simulink subsystem "StudentTemplate_SNGKHA008_M2_Prac"  (R2025b)
settings: Solver=VariableStepAuto  StartTime=0.0  StopTime=10.0  RelTol=1e-3
libraries: simulink x5
settings Model: Creator=JesseJabezArendse  LastModifiedBy=muner

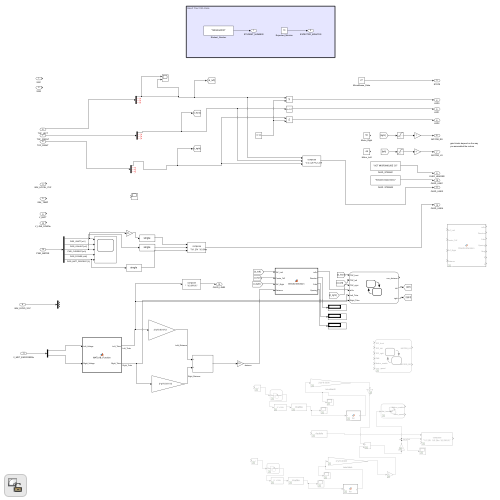
[thumbnail: Simulink's stored preview of the top-level diagram]
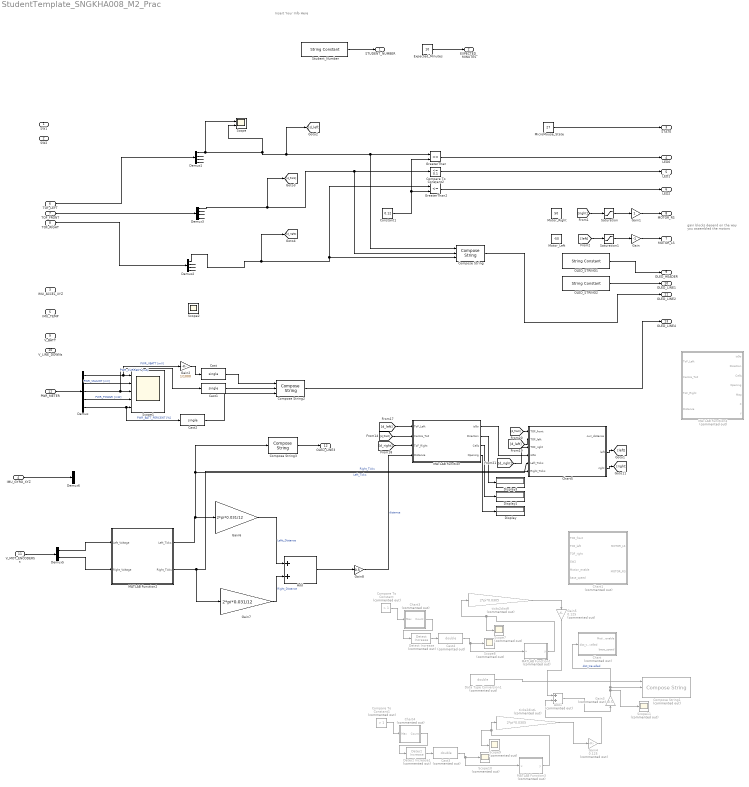
== system StudentTemplate_SNGKHA008_M2_Prac ==
  note: gain blocks depend on the way
      | you assembled the motors
  note: Insert Your Info Here
  SW1 : Inport
  SW2 : Inport  Port=2
  IMU_ACCEL_XYZ : Inport  Port=3
  IMU_GYRO_XYZ : Inport  Port=4
  IMU_TEMP : Inport  Port=5
  TOF_LEFT : Inport  Port=6
  TOF_FRONT : Inport  Port=7
  TOF_RIGHT : Inport  Port=8
  V_BATT : Inport  Port=9
  V_LINE_DOWNs : Inport  Port=10
  V_MOT_ENCODERSs : Inport  Port=11
  PWR_METER : Inport  Port=12
  Add : Sum
  Add1 : Sum  Commented=on
  Cast : DataTypeConversion  OutDataTypeStr=single  SaturateOnIntegerOverflow=off  RndMeth=Floor
  Cast1 : DataTypeConversion  OutDataTypeStr=single  SaturateOnIntegerOverflow=off  RndMeth=Floor
  Cast2 : DataTypeConversion  OutDataTypeStr=single  SaturateOnIntegerOverflow=off  RndMeth=Floor
  Cast3 : DataTypeConversion  Commented=on  OutDataTypeStr=double  SaturateOnIntegerOverflow=off  RndMeth=Floor
  Cast4 : DataTypeConversion  Commented=on  OutDataTypeStr=double  SaturateOnIntegerOverflow=off  RndMeth=Floor
  Chart : Stateflow chart  Commented=on  TreatAsAtomicUnit=on
  Chart1 : Stateflow chart  Commented=on  TreatAsAtomicUnit=on
  Chart3 : Stateflow chart  Commented=on  TreatAsAtomicUnit=on
  Chart4 : Stateflow chart  Commented=on  TreatAsAtomicUnit=on
  Chart5 : Stateflow chart  TreatAsAtomicUnit=on
  Compare To Constant : simulink/Logic and Bit Operations/Compare To Constant  Commented=on  relop=>  const=1  OutDataTypeStr=boolean
  Compare To Constant1 : simulink/Logic and Bit Operations/Compare To Constant  Commented=on  relop=>  const=1  OutDataTypeStr=boolean
  Compare To Constant2 : simulink/Logic and Bit Operations/Compare To Constant  relop=<=  const=0.1  OutDataTypeStr=boolean
  Compose String : ComposeString  Format="\"L%1.2f F%1.2f R%1.2f\""
  Compose String1 : ComposeString  Commented=on  Format="\"%1.2fV  %3.2fm  %2.0f%%\""
  Compose String2 : ComposeString  Format="\"%1.2fV  %3.0fmA  %2.0f%%\""
  Compose String3 : ComposeString  Format="\"  %3.0f%%\""
  Constant1 : Constant  Value=0.12  SampleTime=-1
  Data Type Conversion1 : DataTypeConversion  Commented=on  OutDataTypeStr=double  SaturateOnIntegerOverflow=off  RndMeth=Floor
  Demux : Demux  Outputs=5
  Demux1 : Demux
  Demux2 : Demux
  Demux3 : Demux
  Demux5 : Demux  Outputs=2
  Demux6 : Demux  Outputs=3
  Detect Increase : simulink/Logic and Bit Operations/Detect Increase  Commented=on  vinit=0.0  OutDataTypeStr=boolean
  Detect Increase1 : simulink/Logic and Bit Operations/Detect Increase  Commented=on  vinit=0.0  OutDataTypeStr=boolean
  Display : Display
  Display1 : Display
  Display3 : Display
  Expected_Minutes : Constant  Value=10  OutDataTypeStr=uint8
  Gain : Gain  Gain=-1  OutDataTypeStr=Inherit: Same as input
  Gain1 : Gain  OutDataTypeStr=Inherit: Same as input
  Gain2 : Gain  Gain=1/1000
  Gain3 : Gain  Commented=on  Gain=0.5
  Gain4 : Gain  Commented=on  Gain=0.125
  Gain5 : Gain  Commented=on  Gain=0.125
  Gain6 : Gain  Gain=2*pi*0.031/12
  Gain7 : Gain  Gain=2*pi*0.031/12
  Gain8 : Gain  Gain=0.5  OutDataTypeStr=double
  GreaterThan : RelationalOperator  Operator=<=  OutDataTypeStr=boolean  RndMeth=Simplest  InputSameDT=off
  GreaterThan2 : RelationalOperator  Operator=<=  OutDataTypeStr=boolean  RndMeth=Simplest  InputSameDT=off
  MATLAB Function : MATLAB Function  TreatAsAtomicUnit=on
  MATLAB Function1 : MATLAB Function  Commented=on  TreatAsAtomicUnit=on
  MATLAB Function2 : MATLAB Function  TreatAsAtomicUnit=on
  MATLAB Function3 : MATLAB Function  Commented=on  TreatAsAtomicUnit=on
  MATLAB Function4 : MATLAB Function  Commented=on  TreatAsAtomicUnit=on
  MicroMouse_State : Constant  Value=27
  Motor_Left : Constant  Value=-50
  Motor_Right : Constant  Value=50
  OLED_STRING1 : StringConstant  String="\"UCT MICROMOUSE '25\""
  OLED_STRING2 : StringConstant  String="\"Simulink Data Demo\""
  Saturation : Saturate  UpperLimit=100  LowerLimit=-100
  Saturation1 : Saturate  UpperLimit=100  LowerLimit=-100
  Scope : Scope  NumInputPorts=2
      settings: ActiveDisplayYMinimum=0.22759  ActiveDisplayYMaximum=0.52326  DataLoggingVariableName=ScopeData5
  Scope1 : Scope  NumInputPorts=5
      settings: ActiveDisplayYMinimum=-437.5  ActiveDisplayYMaximum=3937.5  DataLoggingVariableName=ScopeData6
  Scope{7..11} (5 alike) : Scope  Commented=on
      Scope10 settings: ActiveDisplayYMinimum=-1.0332830006305334  ActiveDisplayYMaximum=1.171716999369468
      Scope11 settings: DataLoggingVariableName=ScopeData12
      Scope7 settings: ActiveDisplayYMinimum=34.194505967509976  ActiveDisplayYMaximum=50.493839833256565  DataLoggingVariableName=ScopeData10
      Scope8 settings: ActiveDisplayYMinimum=-1.0332830006305334  ActiveDisplayYMaximum=1.171716999369468  DataLoggingVariableName=ScopeData11
      Scope9 settings: ActiveDisplayYMinimum=34.194505967509976  ActiveDisplayYMaximum=50.493839833256565  DataLoggingVariableName=ScopeData2
  Scope2 : Scope
  Student_Number : StringConstant  String="\"SNGKHA008\""
  ticks2distL : Gain  Commented=on  Gain=2*pi*0.0305
  ticks2distR : Gain  Commented=on  Gain=2*pi*0.0305
  STUDENT_NUMBER : Outport
  EXPECTED_MINUTES : Outport  Port=2
  STATE : Outport  Port=3
  LED0 : Outport  Port=4
  LED1 : Outport  Port=5
  LED2 : Outport  Port=6
  MOTOR_LS : Outport  Port=7
  MOTOR_RS : Outport  Port=8
  OLED_HEADER : Outport  Port=9
  OLED_LINE1 : Outport  Port=10
  OLED_LINE2 : Outport  Port=11
  OLED_LINE3 : Outport  Port=12
  OLED_LINE4 : Outport  Port=13
  wires:
  TOF_FRONT/1 -> Demux3/1
  OLED_STRING2/1 -> OLED_LINE1/1
  Demux2/3 -> ?
  Demux2/2 -> ?
  Demux2/4 -> ?
  Compare To Constant2/1 -> LED1/1
  Demux3/3 -> ?
  TOF_RIGHT/1 -> Demux2/1
  Demux3/4 -> ?
  Demux3/2 -> ?
  Demux1/2 -> ?
  OLED_STRING1/1 -> OLED_HEADER/1
  Compose String/1 -> OLED_LINE2/1
  Constant1/1 -> GreaterThan2/2, GreaterThan/2
  Demux1/4 -> ?
  TOF_LEFT/1 -> Demux1/1
  Demux1/3 -> ?
  PWR_METER/1 -> Demux/1
  Demux/1 -> Scope1/1, Gain2/1  "PWR_VBATT [mV]"
  Demux/2 -> Scope1/2  "PWR_VSHUNT [mV]"
  Demux/3 -> Scope1/3, Cast1/1  "PWR_CURRENT [mA]"
  Demux/4 -> Scope1/4  "PWR_POWER [mW]"
  Demux/5 -> Scope1/5, Cast2/1  "PWR_BATT_PERCENT [%]"
  Compose String2/1 -> OLED_LINE4/1
  Gain2/1 -> Cast/1
  Cast/1 -> Compose String2/1
  Cast1/1 -> Compose String2/2
  Cast2/1 -> Compose String2/3
  Demux2/1 -> Compose String/3, GreaterThan2/1, [d_right]
  Demux1/1 -> Scope/1, Scope/2, Compose String/1, GreaterThan/1, [d_left]
  MicroMouse_State/1 -> STATE/1
  Student_Number/1 -> STUDENT_NUMBER/1
  Expected_Minutes/1 -> EXPECTED_MINUTES/1
  V_MOT_ENCODERSs/1 -> Demux5/1
  [right] -> Saturation/1
  [left] -> Saturation1/1
  IMU_GYRO_XYZ/1 -> Demux6/1
  GreaterThan/1 -> LED0/1
  GreaterThan2/1 -> LED2/1
  Saturation/1 -> Gain1/1
  Saturation1/1 -> Gain/1
  Gain1/1 -> MOTOR_RS/1
  Gain/1 -> MOTOR_LS/1
  Demux3/1 -> Compose String/2, Compare To Constant2/1, [d_front]
  [d_front] -> MATLAB Function/2(Centre_ToF)
  [d_left] -> MATLAB Function/1(ToF_Left)
  [d_right] -> MATLAB Function/3(ToF_Right)
  Demux5/1 -> MATLAB Function2/1(Left_Voltage)
  Demux5/2 -> MATLAB Function2/2(Right_Voltage)
  Add/1 -> Gain8/1
  Gain6/1 -> Add/1  "Leftt_Distance"
  Gain7/1 -> Add/2  "Right_Distance"
  MATLAB Function2/1(Left_Ticks) -> Gain6/1, Chart5/5(Left_Ticks), Compose String3/1  "Left_Ticks"
  MATLAB Function2/2(Right_Ticks) -> Gain7/1, Chart5/6(Right_Ticks)  "Right_Ticks"
  Gain8/1 -> MATLAB Function/4(Distance)  "distance"
  MATLAB Function/1(isGo) -> Chart5/4(isGo)
  [d_left] -> Chart5/2(TOF_left)
  [d_front] -> Chart5/1(TOF_front)
  [d_right] -> Chart5/3(TOF_right)
  Chart5/3(right) -> [right]
  Chart5/2(left) -> [left]
  MATLAB Function/2(Direction) -> Display3/1
  MATLAB Function/3(Cells) -> Display1/1
  MATLAB Function/4(Opening) -> Display/1
  Compose String3/1 -> OLED_LINE3/1
  Cast3/1 -> MATLAB Function3/1(u), Scope10/1
  MATLAB Function3/1(y) -> Scope9/1, ticks2distL/1
  Add1/1 -> Gain3/1
  MATLAB Function1/1(y) -> Scope7/1, ticks2distR/1
  Gain3/1 -> Chart/1(dist_travelled), Compose String1/2, Scope11/1  "dist_travelled"
  Data Type Conversion1/1 -> Compose String1/1
  Compare To Constant1/1 -> Chart4/1(Max)
  Chart4/1(Count) -> Detect Increase1/1
  Chart3/1(Count) -> Detect Increase/1
  Compare To Constant/1 -> Chart3/1(Max)
  Detect Increase/1 -> Cast4/1
  Gain4/1 -> Add1/2
  Gain5/1 -> Add1/1
  Detect Increase1/1 -> Cast3/1
  ticks2distR/1 -> Gain5/1
  Cast4/1 -> MATLAB Function1/1(u), Scope8/1
  ticks2distL/1 -> Gain4/1

== matlab function StudentTemplate_SNGKHA008_M2_Prac/MATLAB Function4 ==
  data: ToF_Left input; isGo output; Centre_ToF input; ToF_Right input; Distance input; Direction output; Cells output; Opening output; Map output; X output; Y output
function [isGo, Direction, Cells, Opening, Map, X, Y] = DirectionDecision(ToF_Left, Centre_ToF, ToF_Right, Distance)
%#codegen
% Determines the robot's movement direction based on ToF sensor readings
% and maps the maze structure.
%
% Outputs a state trigger 'isGo' for a Stateflow chart.
% Also tracks the current facing direction, cell count, and maze map.
%
% Inputs:
%   ToF_Left, Centre_ToF, ToF_Right : Time-of-Flight sensor readings
%   Distance : Total distance traveled (for cell counting)
%
% Outputs:
%   isGo : Numeric trigger for Stateflow
%       1  -> Straight (Start)
%       2  -> Left Turn (turnleft)
%       3  -> Right Turn (turnright)
%       4  -> U-Turn (uturn)
%   Direction : Numeric value representing current facing direction
%       1  -> North
%       2  -> East  
%       3  -> South
%       4  -> West
%   Cells : Number of visited cells
%   Opening : Opening detection
%       -1  -> Opening on left
%       1   -> Opening on right
%       0   -> No opening detected
%   Map : The maze map (Y, X, Layer)
%         Layer 1: North Wall (0=Unk, 1=Wall, 2=Open)
%         Layer 2: East Wall
%         Layer 3: South Wall
%         Layer 4: West Wall
%         Layer 5: Visited (0=No, 1=Yes)
%   X, Y : Robot's current cell coordinates

% --- Thresholds ---
front_threshold = 0.12;
side_threshold  = 0.12;
opening_threshold = 0.2;  % Threshold for detecting openings
cell_distance = 0.16;     % Assumed distance per cell (meters)
post_turn_dist = 0.10;    % Distance to move after turn to center in cell

% --- Map & Coordinate Constants ---
MAP_SIZE_Y = 30;
MAP_SIZE_X = 30;
WALL_N = 1;
WALL_E = 2;
WALL_S = 3;
WALL_W = 4;
LAYER_VISITED = 5;
MAP_UNKNOWN = 0;
MAP_WALL = 1;
MAP_OPEN = 2;

% --- Persistent variables for state tracking ---
persistent currentDirection lastTurnState
persistent lastDistance distanceOffset
persistent lastOpening
persistent startupTimer startupDelayCompleted
persistent postTurnCooldownDistance

% --- NEW Persistent Map & Coordinate variables ---
persistent mazeMap currentX currentY

% --- Initialize persistent variables ---
if isempty(currentDirection)
    currentDirection = 1; % start facing North
    lastTurnState = 0; % previous turn (0 means no-turn)
    
    lastDistance = Distance;
    distanceOffset = Distance; % Initialize offset to current distance
    
    lastOpening = 0; % Initialize opening to 0
    
    startupTimer = 0; % Initialize startup timer
    startupDelayCompleted = false; % Startup delay not completed
    
    postTurnCooldownDistance = 0.0; % Initialize cooldown to 0
    
    % --- NEW Map Initialization ---
    mazeMap = zeros(MAP_SIZE_Y, MAP_SIZE_X, 5, 'uint8');
    currentX = 15; % Start in middle
    currentY = 15; % Start in middle
    % Mark starting cell as visited
    mazeMap(currentY, currentX, LAYER_VISITED) = 1;
end

% --- Startup Delay Logic ---
if ~startupDelayCompleted
    startupTimer = startupTimer + 1;
    if startupTimer >= 100  % Adjust as needed
        startupDelayCompleted = true;
    end
    
    isGo = 0; % Stay still during startup
    Direction = currentDirection;
    Cells = 0;
    Opening = 0;
    % Output initial map and coords
    Map = mazeMap;
    X = currentX;
    Y = currentY;
    return; % Exit early during startup delay
end

% --- NEW: Update Map for CURRENT Cell ---
% This function updates the walls of the cell (currentY, currentX)
% based on the robot's current direction and sensor readings.
mazeMap = updateCellWalls(mazeMap, currentY, currentX, currentDirection, ...
    ToF_Left, Centre_ToF, ToF_Right, ...
    front_threshold, side_threshold, opening_threshold, ...
    MAP_UNKNOWN, MAP_WALL, MAP_OPEN, ...
    WALL_N, WALL_E, WALL_S, WALL_W);

% --- Decide Turn based on sensors ---
opening_left = (ToF_Left > opening_threshold);
opening_right = (ToF_Right > opening_threshold);
localTurn = 0;
if (Centre_ToF < front_threshold) && (ToF_Left < side_threshold) && (ToF_Right < side_threshold)
    localTurn = 2; % dead-end -> U-turn
elseif (Centre_ToF < front_threshold) && (ToF_Left < side_threshold)
    localTurn = 1; % front+left blocked -> turn right
elseif (Centre_ToF < front_threshold) && (ToF_Right < side_threshold)
    localTurn = -1; % front+right blocked -> turn left
elseif (Centre_Tof < front_threshold)
    if ToF_Left > ToF_Right
        localTurn = -1; % more space on left -> turn left
    else
        localTurn = 1;  % more space on right -> turn right
    end
else
    % Front is OPEN (Centre_ToF >= front_threshold)
    
    % Check if we are in the post-turn cooldown period
    if Distance < postTurnCooldownDistance
        % If yes, FORCE straight to clear the corner
        localTurn = 0;
    else
        % If no cooldown, check for side openings as normal
        if opening_left && opening_right
            if ToF_Left > ToF_Right
                localTurn = -1; % Prefer left
            else
                localTurn = 1;  % Prefer right
            end
        elseif opening_left
            localTurn = -1; % Only left is open, turn left
        elseif opening_right
            localTurn = 1;  % Only right is open, turn right
        else
            localTurn = 0; % No openings, go straight
        end
    end
end

% --- Opening Detection Logic ---
if localTurn == 0
    if opening_left
        lastOpening = -1;
    elseif opening_right
        lastOpening = 1;
    else
        lastOpening = 0;
    end
end
Opening = lastOpening;

% --- Update direction only on the rising edge of a turn ---
if (lastTurnState == 0) && (localTurn ~= 0)
    if localTurn == 1
        delta = 1;  % Right turn
    elseif localTurn == -1
        delta = -1; % Left turn
    elseif localTurn == 2
        delta = 2;  % U-turn
    else
        delta = 0;
    end
    currentDirection = mod((currentDirection - 1) + delta, 4) + 1;
end

% --- MODIFIED BLOCK (Handle Cell Transition after a Turn) ---
% Check if we just completed a turn (transition from non-zero to zero)
if (lastTurnState ~= 0) && (localTurn == 0)
    
    % --- NEW: Update Coordinates ---
    % We have finished a turn and are now entering a new cell
    if lastTurnState ~= 2  % If the last turn was NOT a U-turn
        switch currentDirection
            case 1 % Facing North
                currentY = currentY - 1;
            case 2 % Facing East
                currentX = currentX + 1;
            case 3 % Facing South
                currentY = currentY + 1;
            case 4 % Facing West
                currentX = currentX - 1;
        end
        % Mark the new cell as visited
        mazeMap(currentY, currentX, LAYER_VISITED) = 1;
    end
    
    % Force robot to move straight after a turn
    % to clear the corner before making new decisions.
    postTurnCooldownDistance = Distance + post_turn_dist;
    
    distanceOffset = Distance;
end
% Update lastTurnState AFTER the "completed turn" check
if localTurn == 0
    lastTurnState = 0;
else
    lastTurnState = localTurn; % remember we are in a turn state
end
Direction = currentDirection;

% -------- Cell transition logic (straight corridors) --------
% Count cells based on distance traveled when moving straight
if localTurn == 0
    % Calculate effective distance (ignoring distance during turns)
    effectiveDistance = Distance - distanceOffset;
    
    % Each ~0.16 meters = 1 cell
    if effectiveDistance >= (cell_distance + 0.01) % Add small buffer
        cellsFromDistance = floor(effectiveDistance / cell_distance);
        
        % --- NEW: Update Coords for each cell ---
        for i = 1:cellsFromDistance
            switch currentDirection
                case 1 % Facing North
                    currentY = currentY - 1;
                case 2 % Facing East
                    currentX = currentX + 1;
                case 3 % Facing South
                    currentY = currentY + 1;
                case 4 % Facing West
                    currentX = currentX - 1;
            end
            % Mark the new cell as visited
            mazeMap(currentY, currentX, LAYER_VISITED) = 1;
        end
        
        % Update offset to account for counted distance
        distanceOffset = distanceOffset + cellsFromDistance * cell_distance;
    end
end
% --- NEW: Update Cell Count Output ---
Cells = sum(mazeMap(:,:,LAYER_VISITED), 'all');

% -------- Map Turn to isGo output for Stateflow --------
if localTurn == 0
    isGo = 1; % Straight
elseif localTurn == -1
    isGo = 2; % Left Turn
elseif localTurn == 1
    isGo = 3; % Right Turn
elseif localTurn == 2
    isGo = 4; % U-Turn
else
    isGo = 1; % Default to Straight
end

lastDistance = Distance;

% --- NEW: Assign final outputs ---
Map = mazeMap;
X = currentX;
Y = currentY;

end


% --- HELPER FUNCTION ---
function mazeMap = updateCellWalls(mazeMap, Y, X, Direction, ...
    ToF_Left, Centre_ToF, ToF_Right, ...
    front_thresh, side_thresh, opening_thresh, ...
    MAP_UNKNOWN, MAP_WALL, MAP_OPEN, ...
    WALL_N, WALL_E, WALL_S, WALL_W)
%#codegen
% This sub-function updates the map for a single cell (Y,X) based on
% current sensor readings and robot direction.

% 1. Determine relative wall status
isFrontWall = (Centre_ToF < front_thresh);
isFrontOpen = (Centre_ToF > opening_thresh); % Use opening_thresh for "open"

isLeftWall = (ToF_Left < side_thresh);
isLeftOpen = (ToF_Left > opening_thresh);

isRightWall = (ToF_Right < side_thresh);
isRightOpen = (ToF_Right > opening_thresh);

% 2. Map relative directions (Front, Left, Right, Back) to
%    absolute wall indices (N, E, S, W)
idxFront = 0;
idxLeft = 0;
idxRight = 0;
idxBack = 0;

switch Direction
    case 1 % Facing North
        idxFront = WALL_N;
        idxLeft = WALL_W;
        idxRight = WALL_E;
        idxBack = WALL_S;
    case 2 % Facing East
        idxFront = WALL_E;
        idxLeft = WALL_N;
        idxRight = WALL_S;
        idxBack = WALL_W;
    case 3 % Facing South
        idxFront = WALL_S;
        idxLeft = WALL_E;
        idxRight = WALL_W;
        idxBack = WALL_N;
    case 4 % Facing West
        idxFront = WALL_W;
        idxLeft = WALL_S;
        idxRight = WALL_N;
        idxBack = WALL_E;
end

% 3. Update the map layer for each wall
% Only update if we have a confident reading (wall or open)
% Otherwise, leave as MAP_UNKNOWN

% Front Wall
if isFrontWall
    mazeMap(Y, X, idxFront) = MAP_WALL;
elseif isFrontOpen
    mazeMap(Y, X, idxFront) = MAP_OPEN;
end

% Left Wall
if isLeftWall
    mazeMap(Y, X, idxLeft) = MAP_WALL;
elseif isLeftOpen
    mazeMap(Y, X, idxLeft) = MAP_OPEN;
end

% Right Wall
if isRightWall
    mazeMap(Y, X, idxRight) = MAP_WALL;
elseif isRightOpen
    mazeMap(Y, X, idxRight) = MAP_OPEN;
end

% Back Wall (the one we came from)
% If it's unknown, mark it as open.
if mazeMap(Y, X, idxBack) == MAP_UNKNOWN
    mazeMap(Y, X, idxBack) = MAP_OPEN;
end

end

== stateflow chart StudentTemplate_SNGKHA008_M2_Prac/Chart ==
  state MoveForward
    entry:
    Motion_enable = true;
    base_speed = 5;
  state Stop
    entry:
    Motion_enable = false;
    base_speed=0;
  (default) -> MoveForward
  MoveForward -> Stop : [dist_travelled>=1.5]
  data: dist_travelled input; Motion_enable output; base_speed output

== stateflow chart StudentTemplate_SNGKHA008_M2_Prac/Chart3 ==
  state Start
    entry:
    Count = 0;
  state Increase
    entry:
    Count = 1;
  (default) -> Start
  Increase -> Start : after(0.2, sec)
  Start -> Increase : [Max==1]
  data: Max input; Count output

== matlab function StudentTemplate_SNGKHA008_M2_Prac/MATLAB Function1 ==
  data: u input; y output

function y = fcn(u)
persistent lastState pulseCounter

% Initialize on first run
if isempty(lastState)
    lastState = false;
    pulseCounter = 0;
end

% Take first element of input
inputVal = u(1);

% Detection threshold
level = 0.5;
aboveLevel = inputVal > level;

% Count only rising transitions
if aboveLevel && ~lastState
    pulseCounter = pulseCounter + 1;
end

% Output current count
y = pulseCounter;

% Update state memory
lastState = aboveLevel;
end

== stateflow chart StudentTemplate_SNGKHA008_M2_Prac/Chart4 ==
  state Start
    entry:
    Count = 0;
  state Increase
    entry:
    Count = 1;
  (default) -> Start
  Increase -> Start : after(0.2, sec)
  Start -> Increase : [Max==1]
  data: Max input; Count output

== matlab function StudentTemplate_SNGKHA008_M2_Prac/MATLAB Function3 ==
  data: u input; y output
function y = fcn(u)
persistent lastState pulseCounter

% Initialize on first run
if isempty(lastState)
    lastState = false;
    pulseCounter = 0;
end

% Take first element of input
inputVal = u(1);

% Detection threshold
level = 0.5;
aboveLevel = inputVal > level;

% Count only rising transitions
if aboveLevel && ~lastState
    pulseCounter = pulseCounter + 1;
end

% Output current count
y = pulseCounter;

% Update state memory
lastState = aboveLevel;
end

== matlab function StudentTemplate_SNGKHA008_M2_Prac/MATLAB Function ==
  settings: sampleTime=0.1
  data: ToF_Left input; isGo output; Centre_ToF input; ToF_Right input; Distance input; Direction output; Cells output; Opening output
function [isGo, Direction, Cells, Opening] = DirectionDecision(ToF_Left, Centre_ToF, ToF_Right, Distance)
%#codegen
% Determines the robot's movement direction based on ToF sensor readings.
% Outputs a state trigger 'isGo' for a Stateflow chart.
% Also tracks the current facing direction and cell count.
%
% Inputs:
%   ToF_Left, Centre_ToF, ToF_Right : Time-of-Flight sensor readings
%   Distance : Total distance traveled (for cell counting)
%
% Outputs:
%   isGo : Numeric trigger for Stateflow
%       1  -> Straight (Start)
%       2  -> Left Turn (turnleft)
%       3  -> Right Turn (turnright)
%       4  -> U-Turn (uturn)
%   Direction : Numeric value representing current facing direction
%       1  -> North
%       2  -> East  
%       3  -> South
%       4  -> West
%   Cells : Number of cells traversed
%   Opening : Opening detection
%       -1  -> Opening on left
%       1   -> Opening on right
%       0   -> No opening detected

    % Thresholds for obstacle detection (in meters)
    front_threshold = 0.12;
    side_threshold  = 0.12;
    opening_threshold = 0.2;  % Threshold for detecting openings
    
    % Persistent variables for state tracking
    persistent currentDirection lastTurnState
    persistent lastDistance cellCount distanceOffset
    persistent lastOpening  % Store last valid opening
    persistent startupTimer startupDelayCompleted % Startup delay variables
    
    % --- NEW ---
    persistent postTurnCooldownDistance % Cooldown based on distance
    
    % Initialize persistent variables
    if isempty(currentDirection)
        currentDirection = 1; % start facing North
    end
    if isempty(lastTurnState)
        lastTurnState = 0; % previous turn (0 means no-turn)
    end
    if isempty(lastDistance)
        lastDistance = Distance;
        cellCount = 0;
        distanceOffset = 0;
    end
    if isempty(lastOpening)
        lastOpening = 0; % Initialize opening to 0
    end
    if isempty(startupTimer)
        startupTimer = 0; % Initialize startup timer
        startupDelayCompleted = false; % Startup delay not completed
    end
    % --- NEW ---
    if isempty(postTurnCooldownDistance)
        postTurnCooldownDistance = 0.0; % Initialize cooldown to 0
    end

    % --- Startup Delay Logic ---
    if ~startupDelayCompleted
        startupTimer = startupTimer + 1;
        if startupTimer >= 100  % Adjust as needed
            startupDelayCompleted = true;
        end
        
        isGo = 0; % 1 = Straight
        Direction = currentDirection;
        Cells = cellCount;
        Opening = 0;
        return; % Exit early during startup delay
    end

    % --- Decide Turn based on sensors ---
    opening_left = (ToF_Left > opening_threshold);
    opening_right = (ToF_Right > opening_threshold);

    localTurn = 0;
    if (Centre_ToF < front_threshold) && (ToF_Left < side_threshold) && (ToF_Right < side_threshold)
        localTurn = 2; % dead-end -> U-turn
    elseif (Centre_ToF < front_threshold) && (ToF_Left < side_threshold)
        localTurn = 1; % front+left blocked -> turn right
    elseif (Centre_ToF < front_threshold) && (ToF_Right < side_threshold)
        localTurn = -1; % front+right blocked -> turn left
    elseif (Centre_ToF < front_threshold)
        if ToF_Left > ToF_Right
            localTurn = -1; % more space on left -> turn left
        else
            localTurn = 1;  % more space on right -> turn right
        end
    else
        % --- MODIFIED BLOCK ---
        % Front is OPEN (Centre_ToF >= front_threshold)
        
        % Check if we are in the post-turn cooldown period
        if Distance < postTurnCooldownDistance
            % If yes, FORCE straight to clear the corner
            localTurn = 0; 
        else
            % If no cooldown, check for side openings as normal
            if opening_left && opening_right
                if ToF_Left > ToF_Right
                    localTurn = -1; % Prefer left
                else
                    localTurn = 1;  % Prefer right
                end
            elseif opening_left
                localTurn = -1; % Only left is open, turn left
            elseif opening_right
                localTurn = 1;  % Only right is open, turn right
            else
                localTurn = 0; % No openings, go straight
            end
        end
    end

    % --- Opening Detection Logic ---
    if localTurn == 0
        if opening_left
            lastOpening = -1;
        elseif opening_right
            lastOpening = 1;
        else
            lastOpening = 0;
        end
    end
    Opening = lastOpening;

    % --- Update direction only on the rising edge of a turn ---
    if (lastTurnState == 0) && (localTurn ~= 0)
        if localTurn == 1
            delta = 1;
        elseif localTurn == -1
            delta = -1;
        elseif localTurn == 2
            delta = 2;
        else
            delta = 0;
        end
        currentDirection = mod((currentDirection - 1) + delta, 4) + 1;
    end
    
    % --- MODIFIED BLOCK ---
    % Check if we just completed a turn (transition from non-zero to zero)
    if (lastTurnState ~= 0) && (localTurn == 0)
        
        % Set the distance-based cooldown timer when a turn completes
        if lastTurnState ~= 2  % If the last turn was NOT a U-turn
            cellCount = cellCount + 1;
        end
        
        % --- NEW ---
        % Force robot to move ~10cm straight after a turn
        % to clear the corner before making new decisions.
        % TUNE THIS VALUE! If it still clips, make it 0.12 or 0.15.
        postTurnCooldownDistance = Distance + 0.10; 
        
        distanceOffset = Distance;
    end

    % Update lastTurnState AFTER the "completed turn" check
    if localTurn == 0
        lastTurnState = 0;
    else
        lastTurnState = localTurn; % remember we are in a turn state
    end
    Direction = currentDirection;
    
    % -------- Cell counting logic (based on distance) --------
    % Count cells based on distance traveled when moving straight
    if localTurn == 0
        % Calculate effective distance (ignoring distance during turns)
        effectiveDistance = Distance - distanceOffset;
        
        % Each ~0.16 meters = 1 cell
        if effectiveDistance >= 0.17
            cellsFromDistance = floor(effectiveDistance / 0.16);
            cellCount = cellCount + cellsFromDistance;
            % Update offset to account for counted distance
            distanceOffset = distanceOffset + cellsFromDistance * 0.16;
        end
    end
    Cells = cellCount;
    
    % -------- Map Turn to isGo output for Stateflow --------
    if localTurn == 0
        isGo = 1; % Straight
    elseif localTurn == -1
        isGo = 2; % Left Turn
    elseif localTurn == 1
        isGo = 3; % Right Turn
    elseif localTurn == 2
        isGo = 4; % U-Turn
    else
        isGo = 1; % Default to Straight
    end
    
    lastDistance = Distance;
end

== stateflow chart StudentTemplate_SNGKHA008_M2_Prac/Chart5 ==
  settings: sampleTime=0.1
  state Stop [commented out]
    entry:
    left = 0;
    right = 0;
  state Turnleft
    entry:
    left = -70;
    right = 70;
    start_ticks_right = Right_Ticks;
    during:
    delta_ticks = abs(Right_Ticks - start_ticks_right);
  state wait
    entry:
    left = 0;
    right = 0;
  state Start
    entry:
    curr_distance = TOF_front;
    correction = calculateSteeringCorrection(TOF_left, TOF_right);
    left = 70   + correction;
    right = 70 - correction;
    during:
    correction = calculateSteeringCorrection(TOF_left, TOF_right);
    left = 70 + correction;
    right = 70 - correction;
  state WaitForTurn_L
    entry:
    left =70;
    right =70;
  state Initialize_straight
    entry:
    left = 0;
    right = 0;
  state MoveCell
    entry:
    left = 0;
    right = 0;
  state Initialize_turn_L
    entry:
    left = 0;
    right = 0;
  state Uturn
    entry:
    left = -70;
    right = 70;
    start_ticks_right = Right_Ticks;
    during:
    delta_ticks = abs(Right_Ticks - start_ticks_right);
  state WaitForTurn_R
    entry:
    left =70;
    right =70;
  state Initialize_turn_R
    entry:
    left = 0;
    right = 0;
  state Turnright
    entry:
    left = 70;
    right = -70;
    start_ticks_left = Left_Ticks;
    during:
    delta_ticks = abs(Left_Ticks - start_ticks_left);
  state WaitForStraight
    entry:
    curr_distance = TOF_front;
    correction = calculateSteeringCorrection(TOF_left, TOF_right);
    left = 70   + correction;
    right = 70 - correction;
    during:
    correction = calculateSteeringCorrection(TOF_left, TOF_right);
    left = 70 + correction;
    right = 70 - correction;
  state wait1
    entry:
    left = 0;
    right = 0;
  wait -> WaitForTurn_L [commented out] : [isGo == 2]
  Stop -> Turnleft [commented out] : [TOF_left > 0.2]
  Start -> Stop [commented out] : [TOF_front <= 0.12]
  Stop -> Uturn [commented out] : [TOF_front<=0.12 && TOF_left<=0.12 && TOF_right <= 0.12 ]
  Stop -> Turnright [commented out] : [TOF_right > 0.2]
  Start -> wait [order 2] : [isGo ~= 1]
  (default) -> wait
  Start -> Turnright [commented out] : [isGo == 3]
  Start -> Turnleft [commented out] : [isGo == 2]
  wait -> Start [commented out] : [isGo == 1]
  wait -> Initialize_straight [order 2] : [isGo ==1]
  WaitForStraight -> wait [commented out] : after(0.015, sec)
  WaitForTurn_L -> Turnleft : after(0.01, sec)
  wait1 -> wait : after(0.015, sec)
  wait -> WaitForTurn_R [commented out] : [isGo == 3]
  wait -> Initialize_turn_R [order 4] : [isGo == 3]
  wait -> Initialize_turn_L [order 3] : [isGo ==2]
  wait -> Uturn [order 1] : [isGo == 4]
  Initialize_turn_L -> WaitForTurn_L : after(0.02, sec)
  Start -> MoveCell [order 1] : after(0.02, sec)
  Initialize_straight -> Start : after(0.01, sec)
  Turnleft -> WaitForStraight : after(0.0095, sec)
  Start -> WaitForStraight [commented out] : after(0.025, sec)
  MoveCell -> Start : after(0.001, sec)
  WaitForStraight -> Start [commented out] : after(0.001, sec)
  Initialize_turn_R -> WaitForTurn_R : after(0.02, sec)
  WaitForTurn_R -> Turnright : after(0.0105, sec)
  Uturn -> WaitForStraight : after(0.02, sec)
  Turnright -> WaitForStraight : after(0.0095, sec)
  WaitForStraight -> wait1 : after(0.02, sec)
  data: left_distance function_input; right_distance function_input; correction function_output; TOF_front input; TOF_left input; TOF_right input; isGo input; curr_distance output; left output; right output; correction local; Left_Ticks input; Right_Ticks input; delta_ticks local; start_ticks_left local; start_ticks_right local; TICK_TARGET_RIGHT constant double =11; TICK_TARGET_LEFT constant double =11
  function correction = calculateSteeringCorrection(left_distance, right_distance):
    | function correction = calculateSteeringCorrection(left_distance, right_distance)
    | %#codegen
    | % CALCULATESTEERINGCORRECTION - Computes steering correction using PD control.
    | %
    | % Inputs:
    | %   left_distance  - Left wall distance in mm (uint32)
    | %   right_distance - Right wall distance in mm (uint32)
    | %   last_error     - Previous steering error (int16)
    | %
    | % Output:
    | %   correction     - Steering correction (int8)
    | %
    | % This block can be used inside Simulink to steer a maze robot or Micromouse.
    | 
    | % Define constants
    | MIN_WALL_DETECT_MM     = 30;     % minimum valid wall distance [mm]
    | MAX_WALL_DETECT_MM     = 120;    % maximum valid wall distance [mm]
    | TARGET_WALL_DISTANCE_MM = 80;   % desired distance from wall [mm]
    | MAX_STEERING_CORRECTION = 30;    % maximum steering correction (deg or motor diff)
    | 
    | % --- Persistent variable for derivative ---
    | persistent last_steering_error
    | if isempty(last_steering_error)
    |     last_steering_error = double(0);
    | end
    | 
    | % Initialize outputs
    | error = double(0);
    | correction = double(0);
    | left_distance = left_distance * 1000;
    | right_distance = right_distance * 1000;
    | % Check which walls are valid
    | left_valid  = (left_distance  >= MIN_WALL_DETECT_MM) && (left_distance  <= MAX_WALL_DETECT_MM);
    | right_valid = (right_distance >= MIN_WALL_DETECT_MM) && (right_distance <= MAX_WALL_DETECT_MM);
    | 
    | % --- Determine error based on wall detection ---
    | if left_valid && right_valid
    |     % Both walls detected – stay centered
    |     left_error  = double(TARGET_WALL_DISTANCE_MM - double(left_distance));
    |     right_error = double(double(right_distance) - TARGET_WALL_DISTANCE_MM);
    |     error = double((double(left_error) + double(right_error)));
    | 
    | elseif left_valid
    |     % Only left wall detected – keep distance from left
    |     error = double(TARGET_WALL_DISTANCE_MM - double(left_distance));
    | 
    | elseif right_valid
    |     % Only right wall detected – keep distance from right
    |     error = double(double(right_distance) - TARGET_WALL_DISTANCE_MM);
    |     %error = error; % invert for correct steering direction
    | 
    | else
    |     % No walls detected – go straight
    |     error = double(0);
    |     last_steering_error = double(0);
    |     correction = double(0);
    |     return;
    | end
    | 
    | % --- PD Control ---
    | derivative = double(error - last_steering_error);
    | 
    | correction_scaled = double((0.5 * 10.0) * double(error) + ...
    |                           (0.3 * 10.0) * double(derivative));
    | 
    | correction_val = correction_scaled / 10;
    | 
    | % --- Update last error ---
    | last_steering_error = error;
    | 
    | % --- Limit correction ---
    | if correction_val > MAX_STEERING_CORRECTION
    |     correction_val = MAX_STEERING_CORRECTION;
    | elseif correction_val < -MAX_STEERING_CORRECTION
    |     correction_val = -MAX_STEERING_CORRECTION;
    | end
    | 
    | correction = double(correction_val);
    | 
    | end

== matlab function StudentTemplate_SNGKHA008_M2_Prac/MATLAB Function2 ==
  settings: updateMethod=DISCRETE
  data: Left_Voltage input; Left_Ticks output; Right_Ticks output; Right_Voltage input
 function [Left_Ticks, Right_Ticks] = MATLAB_Function(Left_Voltage, Right_Voltage)

    Right_Voltage = single(Right_Voltage) %Voltage measured from right wheel
    Left_Voltage = single( Left_Voltage)  %Voltage measured from left wheel
    persistent prev_right prev_left right_count left_count % Prevous count variables
    if isempty(prev_right)   % countering for empty variables
        prev_right   = single(0);
        prev_left    = single(0);
        right_count  = single(0);
        left_count   = single(0);
    end

    if prev_right < single(1.9) && Right_Voltage > single(1.9)  % Change will occr at 1 as I muliplied it by 2
    right_count = right_count + single(1);
    end

    if prev_left < single(1.3) && Left_Voltage > single(1.3)
        left_count = left_count + single(1);
    end

    prev_right = Right_Voltage;
    prev_left  = Left_Voltage;

    Right_Ticks = right_count;
    Left_Ticks  = left_count;
end

== stateflow chart StudentTemplate_SNGKHA008_M2_Prac/Chart1 ==
  state Idle
    entry:
    MOTOR_LS = 0;
    MOTOR_RS = 0;
  state LeftCorrection
    entry:
    MOTOR_LS =base_speed- 50;
    MOTOR_RS = base_speed;
  state Start
    entry:
    MOTOR_LS = base_speed;
    MOTOR_RS = base_speed;
  state IgnoreRight
    entry:
    MOTOR_LS = base_speed-10;
    MOTOR_RS = base_speed;
  state RghtCorrection
    entry:
    MOTOR_LS = base_speed;
    MOTOR_RS = base_speed - 50;
  state IgnoreLeft
    entry:
    MOTOR_LS = base_speed;
    MOTOR_LS = base_speed-10;
  state FullTurn
    entry:
    MOTOR_LS = base_speed;
    MOTOR_RS = -base_speed;
  IgnoreRight -> Idle [order 2] : [Motion_enable==false]
  IgnoreLeft -> Idle [order 2] : [Motion_enable==false]
  LeftCorrection -> Idle [order 5] : [Motion_enable==false]
  LeftCorrection -> IgnoreLeft [order 2] : [TOF_left - TOF_right>0.1]
  IgnoreLeft -> LeftCorrection [order 1] : after(0.2, sec)
  (default) -> Idle
  LeftCorrection -> IgnoreRight [order 3] : [TOF_left - TOF_right<-0.1]
  Start -> Idle [order 3] : [Motion_enable==false]
  RghtCorrection -> Idle [order 5] : [Motion_enable==false]
  FullTurn -> Idle [order 2] : [Motion_enable==false]
  Start -> LeftCorrection [order 1] : [TOF_left-TOF_right<0]
  LeftCorrection -> FullTurn [order 1] : [TOF_front<0.1 && (TOF_left - TOF_right < 0 || TOF_left - TOF_right > 0)]
  LeftCorrection -> RghtCorrection [order 4] : [TOF_left-TOF_right]
  RghtCorrection -> LeftCorrection [order 4] : [TOF_left-TOF_right]
  Idle -> Start : [SW2==0 && Motion_enable == true]
  IgnoreRight -> RghtCorrection [order 1] : after(0.2, sec)
  RghtCorrection -> IgnoreRight [order 3] : [TOF_left-TOF_right<-0.1]
  Start -> RghtCorrection [order 2] : [TOF_left - TOF_right>0]
  FullTurn -> RghtCorrection [order 1] : [TOF_front<0.1 && (TOF_left - TOF_right <0 || TOF_left - TOF_right > 0)]
  RghtCorrection -> FullTurn [order 1] : [TOF_right<0.1]
  RghtCorrection -> IgnoreLeft [order 2] : [TOF_left-TOF_right>0.1]
  data: TOF_front input; TOF_left input; TOF_right input; MOTOR_LS output; MOTOR_RS output; SW2 input; Motion_enable input; base_speed input
